simulink subsystem "NV_memristor_Simulink"  (R2025b)
settings: Solver=VariableStepAuto  StartTime=0.0  StopTime=10.0  RelTol=1e-3
settings Model: DefaultTestHarness=Memristor_NonVolatile_Subsystem_Harness1  Creator=georg  LastModifiedBy=chipher

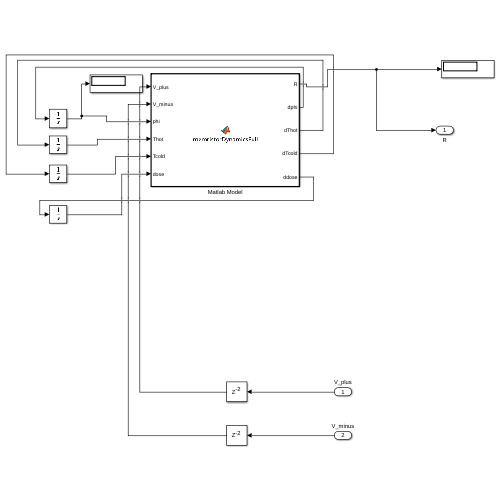
[thumbnail: Simulink's stored preview of the top-level diagram]
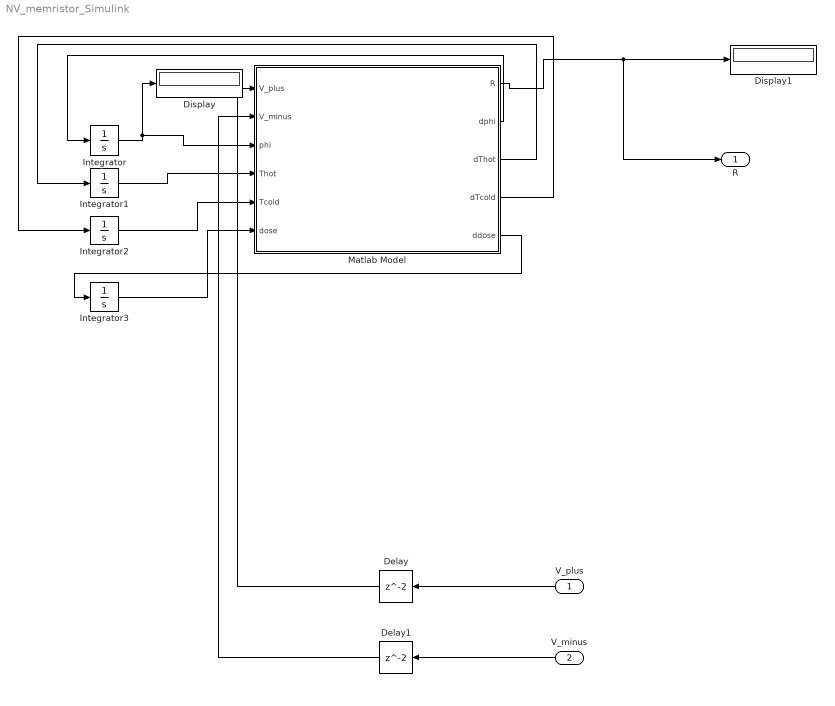
== system NV_memristor_Simulink ==
  V_plus : Inport
  V_minus : Inport  Port=2
  Delay : Delay
  Delay1 : Delay
  Display : Display
  Display1 : Display
  Integrator : Integrator  InitialCondition=6e-09
  Integrator1 : Integrator  InitialCondition=300
  Integrator2 : Integrator  InitialCondition=300
  Integrator3 : Integrator
  Matlab Model : MATLAB Function  TreatAsAtomicUnit=on
  R : Outport  VectorParamsAs1DForOutWhenUnconnected=off
  wires:
  Matlab Model/2(dphi) -> Integrator/1
  Integrator1/1 -> Matlab Model/4(Thot)
  Matlab Model/3(dThot) -> Integrator1/1
  Matlab Model/4(dTcold) -> Integrator2/1
  Matlab Model/5(ddose) -> Integrator3/1
  Integrator2/1 -> Matlab Model/5(Tcold)
  Integrator3/1 -> Matlab Model/6(dose)
  Integrator/1 -> Matlab Model/3(phi), Display/1
  Matlab Model/1(R) -> R/1, Display1/1
  V_plus/1 -> Delay/1
  Delay/1 -> Matlab Model/1(V_plus)
  V_minus/1 -> Delay1/1
  Delay1/1 -> Matlab Model/2(V_minus)

== matlab function NV_memristor_Simulink/Matlab Model ==
  data: V_plus input; V_minus input; R output; phi input; Thot input; Tcold input; dphi output; dThot output; dTcold output; dose input; ddose output
function [R, dphi, dThot, dTcold, ddose] = memristorDynamicsFull(V_plus, V_minus, phi, Thot, Tcold, dose)
% Inputs: voltage terminals, state variables (phi, Thot, Tcold, dose)
% Outputs: resistance R, and derivatives of each state variable

% === Voltage ===
V = V_plus - V_minus;

%% Parameters

params = struct(...
    'q',                1.602176634e-19, ...
    'kb',               1.38064852e-23, ...
    'rT',               20e-9, ...
    'rB',               4e-9, ...
    'L',                20e-9, ...
    'g',                1e-9, ...
    'phi_max',          12e-9, ...
    'phi_min',          0.01e-9, ...
    'Tamb',             300, ... 
    'Tau_th',           2.3e-9, ...
    'm',                2000e-9, ...
    'rbulkm',           3e-13, ...
    'rbulkox',          1000, ...
    'gamma',            20e-9, ...
    'el',               28e-9, ...
    'p',                0.5, ...
    'AP',               1.5, ...
    'BP',               1e-4, ...
    'CP',               1.2e-24, ...
    'Edrift',           1.15 * 1.602176634e-19, ...
    'Ediff',            2.5 * 1.602176634e-19, ...
    'alphaP',           1.0, ...
    'Aexp',             0.5, ...
    'Es',               0.8 * 1.602176634e-19, ...
    'phi_sat',          2e-9, ...
    'phi_B',            0.65 * 1.602176634e-19, ...
    'A_star',           1.2e6, ...
    'n_schottky',       1.5, ...
    'lambda_plasticity',200, ...
    'gamma_dose',       1, ...
    'T_trigger',        400, ...
    'T_slope',          20, ...
    'Vmax',             30, ...
    'Km',               1e-15, ...
    'healing_rate',     1 ...
);




% --- Unpack model parameters from struct --- Getting lazy!
q     = params.q;
kb    = params.kb;
rT    = params.rT;
rB    = params.rB;
L     = params.L;
g     = params.g;
phi_max = params.phi_max;
phi_min = params.phi_min;
Tamb  = params.Tamb;
Tau_th = params.Tau_th;
m     = params.m;
rbulkm = params.rbulkm;
rbulkox = params.rbulkox;
gamma  = params.gamma;
el    = params.el;
p     = params.p;
AP    = params.AP;
BP    = params.BP;
CP    = params.CP;
Edrift = params.Edrift;
Ediff  = params.Ediff;
alphaP = params.alphaP;
Aexp  = params.Aexp;
Es    = params.Es;
phi_sat = params.phi_sat;
phi_B = params.phi_B;
A_star = params.A_star;
n_schottky = params.n_schottky;
lambda_plasticity = params.lambda_plasticity;
gamma_dose = params.gamma_dose;
T_trigger = params.T_trigger;
T_slope = params.T_slope;
Vmax  = params.Vmax;
Km    = params.Km;
healing_rate = params.healing_rate;
%phi_switch = params.phi_switch;

% Utilities
st_f = @(y, y0) 1 ./ (1 + exp(-y ./ y0));
soft_barrier = @(y, width) 1 ./ (1 + (y ./ width).^2);

% Compute values
S = Es / (kb * Thot^2);
E = V / g;

rx1 = rT - ((rT - phi/2) / (L/2)) * ((L/2) - g);
rx2 = rB - ((rB - phi/2) / (L/2)) * ((L/2) - g);
rcf = rbulkm * (1 + (3/4)*(el/phi)*(1 - p));
rox = rbulkox / (1 + gamma*abs(E));
Roff = (rcf*(L-g)/(2*pi*rT*rx1)) + ...
       (rcf*(L-g)/(2*pi*rB*rx2)) + ...
       (rox * g / (pi * rx1 * rx2));
Ron = (rcf * L / (2*pi*rT*phi/2)) + ...
      (rcf * L / (2*pi*rB*phi/2));
R = st_f(phi - phi_max, 1e-9).*Ron + ...
    st_f(phi_min - phi, 1e-9).*Roff;

% === Currents ===
phi_limit = 0.2e-9;
Area_eff = pi * (min(phi, phi_limit)/2)^2;
J0 = A_star * Thot^2 * exp(-phi_B / (kb * Thot));
J_schottky = J0 * (1-exp(-q*V / (n_schottky*kb*Thot)) );
I_schottky = J_schottky * Area_eff;
I_cf = V / R;
I_total = I_cf + I_schottky;

% === Thermal dynamics ===
kthcold = m * (2 * rT);
kthhot = m * phi;
dTcold = (abs(V * I_total) / kthcold + Tamb / Tau_th - Tcold / Tau_th);
dThot  = (abs(V * I_total) / kthhot + Tamb / Tau_th - Thot / Tau_th);
deltaT = Thot - Tcold;
T = Thot;

% === Filament dynamics ===
drift = AP * exp(-Aexp * (Edrift - alphaP * q * V) / (kb * T)) * st_f(V, 0.2) * soft_barrier(phi - phi_max, 1e-5);
diff = BP * (1/phi) * exp(-Ediff / (kb*T)) * (1 + gamma_dose*dose) * exp(-phi / phi_sat);
thermal = CP * S * (1/phi) * deltaT / (L/2) * (1 + lambda_plasticity * dose);
thermal = thermal * (1 + (0.5 + 0.5*tanh((deltaT - T_trigger) / T_slope)));
neg_drift = AP * exp(-Aexp * (Edrift - alphaP*q*abs(V)) / (kb*T)) * ...
            st_f(-V, 0.2) * st_f(phi - phi_max, 1e-9);

dphi = st_f(phi_max - phi, 1e-9) * (drift + diff - thermal) - ...
       st_f(phi - phi_min, 1e-9) * (diff + neg_drift + thermal);


% Wall steepness (controls how "hard" the wall is)
wall_stiffness = 1e16; 

% 1. Detect if we are pushing against a wall
% pushing_bottom is 1 if phi < phi_min AND dphi is negative
pushing_bottom = (0.5 + 0.5 * tanh((phi_min - phi) * wall_stiffness)) .* ...
                 (0.5 + 0.5 * tanh(-dphi * wall_stiffness));

% pushing_top is 1 if phi > phi_max AND dphi is positive
pushing_top    = (0.5 + 0.5 * tanh((phi - phi_max) * wall_stiffness)) .* ...
                 (0.5 + 0.5 * tanh(dphi * wall_stiffness));

% 2. Apply the brakes
% If pushing against a wall, multiply dphi by 0. Otherwise multiply by 1.
wall_factor = (1 - pushing_bottom) * (1 - pushing_top);

dphi = dphi * wall_factor;

% Dose dynamics
absorbed_energy = abs(V * I_total);
temperature_factor = max((T - Tamb), 0) / Tamb;
%dose_rate = (Vmax * absorbed_energy * temperature_factor) / ...
            %(Km + absorbed_energy * temperature_factor);
V_thresh = 0.1;
polarity_gate = 1 / (1 + exp(-V / V_thresh));  % V_thresh ~ 0.05 V
dose_rate = polarity_gate * (Vmax * absorbed_energy * temperature_factor) / ...
            (Km + absorbed_energy * temperature_factor);

healing_effect = exp(-(Tcold - Tamb) / 10);
ddose = dose_rate - healing_rate * healing_effect * dose;

end
